simulink model "Gesamtmodell_Umbenannt"  (R2017b)
settings: Solver=ode3  StartTime=0.0  StopTime=inf  FixedStep=dt  RelTol=1e-3  EnableMultiTasking=on
InitFcn:
  | Reglerauslegung
undefined symbols (not defined in the file or in its folder): aMax, aMaxPsi, Blindzeit, Com1, dt, K1, K2, K3, Kx, Ky, none, sigbuilder_block, Tx, Ty, vMax, vMaxPsi
libraries: xpcrtudplib x11, simulink x6, xpcutilitieslib x4, xpcseriallib x1, slrtlib x1
(part 4 of 4)

== matlab function Gesamtmodell_Umbenannt/Regelung1/Zustandsautomat/KoordonatenTafel1 ==
  data: stationsNr input; zielX output; zielY output; zielPsi output; toleranzStufe output; StationsKoordinaten parameter; enable output; Korrektur input
function [zielX, zielY, zielPsi, toleranzStufe, enable] = koordinaten(stationsNr,StationsKoordinaten,Korrektur)

xBuchtOffset = 10;
% 1 -> genau, 2 -> ungenau
toleranzStufe = 1;
enable = 1;

% Batteriestationen anfahren

if stationsNr == 80
    zielX   = StationsKoordinaten(1,stationsNr);
    zielY   = StationsKoordinaten(2,stationsNr);
    zielPsi = pi;
    return
end

if stationsNr == 90
    zielX   = StationsKoordinaten(1,stationsNr);
    zielY   = StationsKoordinaten(2,stationsNr);
    zielPsi = pi;
    return
end

if stationsNr == 100
    zielX   = StationsKoordinaten(1,stationsNr);
    zielY   = StationsKoordinaten(2,stationsNr);
    zielPsi = pi;
    return
end

if stationsNr == 110
    zielX   = StationsKoordinaten(1,stationsNr);
    zielY   = StationsKoordinaten(2,stationsNr);
    zielPsi = pi;
    return
end

% Warteposition vorne
if mod(stationsNr, 10) == 0 
    toleranzStufe = 2;
    
        % WartePosition 0
        if stationsNr == 0
            %weil Matlab leider nicht von 0 aus zählen kann müssen wir das von
            %Hand abfangen...doofes Matlab
            zielX   = 853;
            zielY   = 2288;
            zielPsi = pi/2;
        else
            zielX   = StationsKoordinaten(1,stationsNr);
            zielY   = StationsKoordinaten(2,stationsNr);
            zielPsi = pi/2;
        end

% Stations-Bucht
elseif 0 < mod(stationsNr, 10) && mod(stationsNr, 10) < 4
    
    zielX   = StationsKoordinaten(1,stationsNr);
    zielY   = StationsKoordinaten(2,stationsNr);
    
    % auf welcher Seite der Station?
    if mod(stationsNr, 20) < 10
        % links
        zielX = zielX + xBuchtOffset+Korrektur *5;
        zielPsi = 0;
    else
        % rechts
        zielX = zielX - xBuchtOffset-Korrektur *5;
        zielPsi = pi;
    end

% Warteposition hinten
elseif mod(stationsNr, 10) == 4
    toleranzStufe = 2;
    
    zielX   = StationsKoordinaten(1,stationsNr);
    zielY   = StationsKoordinaten(2,stationsNr);
    zielPsi = pi/2;

% Warteposition mitte
elseif mod(stationsNr, 10) == 5
    
    zielX   = StationsKoordinaten(1,stationsNr);
    zielY   = StationsKoordinaten(2,stationsNr);
    zielPsi = pi/2;

% Vorposition der Bucht
elseif 5 < mod(stationsNr, 10) && mod(stationsNr, 10) < 9
    
    % auf welcher Seite der Station?
    if mod(stationsNr, 20) < 10
        % links
        zielX   = StationsKoordinaten(1,stationsNr-5) - 100;
        zielY   = StationsKoordinaten(2,stationsNr-5);
        zielPsi = 0;
    else
        % rechts
        zielX   = StationsKoordinaten(1,stationsNr-5) + 100;
        zielY   = StationsKoordinaten(2,stationsNr-5);
        zielPsi = pi;
    end

% eine nicht zugeteilte Stationsnummer wird angefordert
else
    % Roboter anhalten
    enable = 0;

    zielX   = 0;
    zielY   = 0;
    zielPsi = 0;
end

== matlab function Gesamtmodell_Umbenannt/Regelung1/Zustandsautomat/zielErreicht ==
  data: roboX input; erreicht output; roboY input; roboPsi input; zielX input; zielY input; zielPsi input; toleranzStufe input
 function erreicht = zielErreicht(roboX, roboY, roboPsi, zielX, zielY, zielPsi, toleranzStufe)

 if( toleranzStufe == 2)
    % ungenau
    transToleranz = 50;
    rotToleranz = pi/2;
 else
    % default = genau
    transToleranz = 15;
    rotToleranz = pi/20;
 end

    erreicht = 0;
    
%     if( TasterGreifer == 1)
%         erreicht = 1;
%         return;
%     end
    
    if( abs(zielX-roboX) > transToleranz)
        return;
    end 
    
    if( abs(zielY-roboY) > transToleranz)
        return;
    end 
       
    if( abs(zielPsi-mod(roboPsi,2*pi)) > rotToleranz)&&( abs(zielPsi+2*pi-mod(roboPsi,2*pi)) > rotToleranz)
        return;
    end   

    erreicht = 1;

end

== matlab function Gesamtmodell_Umbenannt/Regelung1/Zustandsregler/Winkelentstoerung ==
  data: Ist input; Soll input; Out output



function Out = Winkel(Ist,Soll)

Ist = mod(Ist, 2*pi);      % Normierung des Ist-Winkels auf das Intervall 0° - 360°
Soll = mod(Soll, 2*pi);    % Normierung des Soll-Winkels auf das Intervall 0° - 360°

if (abs(Soll-Ist) <= pi)   % (1)
    
    Out = Soll - Ist;      % (2)
    
else
    
     if (Soll > Ist)                % (3)
        Out = Soll - Ist - 2*pi;    % (4)
     else
         Out = Soll - Ist + 2*pi;   % (5)
     end
end

% Problem: 
% Beim Durchschreiten der Grenze 0°/360° entsteht ein Sprung in
% der Regeldifferenz beim Winkel, der zu einer unkontrollierten Rotation
% des Robotino führt
% 
% Lösung: 
% Impelementierung einer Fallunterscheidung, die die tatsächliche
% Regeldifferenz unter Berücksichtigung der Grenze 0°/360° ausgibt
% 
% Ansatz: 
% Prüfung, ob die vorgegebene Trajektorie über die kritische Grenze
% führt (1). Führt die Trajektorie über die kritische Grenze, ist
% der Betrag der Differenz zwischen Soll- und Istwert > pi.
% 
% Bei unkritischen Trajektorien wird die Regeldifferenz über die Formel (2)
% zurückgegeben.
%
% Bei kritischen Trajektorien muss zuerst unterschieden werden, in welchem
% Drehsinn die kritische Grenze durchschritten wird (3). Bei positivem
% Drehsinn wird die Differenz nach Formel (4) ermittelt, bei negativem
% Drehsinn wird die Differenz nach Formal (5) ermittelt. 
%
% Die Ausgabe der Regeldifferenz erfolgt immer in Richtung und Betrag, bei
% einem positiven Vorzeichen befindet sich die Sollposition in mathematisch
% positivem Drehsinn, bei einem negativen Vorzeichen befindet sie sich in
% mathematisch negativem Drehsinn. Der Betrag gibt die verbleibene
% Winkeldifferenz zur Sollposition an.

== matlab function Gesamtmodell_Umbenannt/Regelung1/enable  ==
  data: BereichsModus input; enableBereich input; enableKamera input; enableBeobachter input; enable output; enableKoord input; enableFlogik input
function enable  = enable(BereichsModus, enableBereich,enableKamera,enableBeobachter,enableKoord,enableFlogik)
    if BereichsModus == 1
        % Fertigungsbereich
        if enableBereich && (enableKamera || enableBeobachter )&& enableKoord && enableFlogik
            enable = 1;
        else 
            enable = 0;
        end
    else
        % Transportbereich
        if enableKamera || enableBeobachter 
            % mindestens kamera oder beobachter muessen funktionieren            
            enable = 1;
        else
            % sonst nix fahren 
            enable = 0;
        end
    end
    
end

== matlab function Gesamtmodell_Umbenannt/Regelung1/u(x,v)  ==
  data: v1 input; v2 input; v3 input; x1 input; x2 input; x3 input; x4 input; u1 output; u2 output; u3 output; Tx parameter; Ty parameter; Kx parameter; Ky parameter
function [u1, u2, u3]= inputLinearisierung(v1,v2,v3,x1,x2,x3,x4,Tx,Ty,Kx,Ky)


%u1 = (Ty*x1 - Tx*x1 + Ty*v1*cos(x4) + Tx*v2*sin(x4) + Tx*x1*cos(x4)^2 - Ty*x1*cos(x4)^2 - (Tx*x2*sin(2*x4))/2 + (Ty*x2*sin(2*x4))/2 + Tx*Ty*x2*x3)/Ty;
%u2 = -(Ty*x2 - Tx*x2 - Tx*v2*cos(x4) + Ty*v1*sin(x4) + Tx*x2*cos(x4)^2 - Ty*x2*cos(x4)^2 + (Tx*x1*sin(2*x4))/2 - (Ty*x1*sin(2*x4))/2 + Tx*Ty*x1*x3)/Tx;
u1 = (Ty*x1 - Tx*x1 + Tx*x1*cos(x4)^2 - Ty*x1*cos(x4)^2 - (Tx*x2*sin(2*x4))/2 + (Ty*x2*sin(2*x4))/2 + Kx*Ty*v1*cos(x4) + Ky*Tx*v2*sin(x4) + Tx*Ty*x2*x3)/(Kx*Ty);
u2 = -(Ty*x2 - Tx*x2 + Tx*x2*cos(x4)^2 - Ty*x2*cos(x4)^2 + (Tx*x1*sin(2*x4))/2 - (Ty*x1*sin(2*x4))/2 - Ky*Tx*v2*cos(x4) + Kx*Ty*v1*sin(x4) + Tx*Ty*x1*x3)/(Ky*Tx);
u3 = v3;

== matlab function Gesamtmodell_Umbenannt/Regelung1/z(x) ==
  data: x1 input; x2 input; x3 input; x4 input; z1 output; z5 output; z2 output; z6 output; x5 input; x6 input; z3 output; z4 output
function [z1,z5,z2,z6,z3,z4]= zustandsTrafo(x1,x2,x3,x4,x5,x6)

z1 = cos(x4) * x1 - sin(x4) * x2;
z2 = sin(x4) * x1 + cos(x4) * x2;
z3 = x3;
z4 = x4;
z5 = x5;
z6 = x6;
